simulink model "Simulink_Sfunc_Sim"  (R2022b)
settings: Solver=FixedStepAuto  StartTime=0.0  StopTime=5  FixedStep=0.01  RelTol=1e-3
values from neighbouring files (symbols this model uses):
  N = 20    [Aircraft_MPC_No_Rate_Constraints.m]    (also in Aircraft_MPC_v1.m = 100)
  nu = model.u.rows()    [Aircraft_MPC_No_Rate_Constraints.m]    (also in Aircraft_MPC_v1.m; get_aircraft_model.m = 4)
  u_max = [20000; 20000; 1700; 1700]    [Aircraft_MPC_No_Rate_Constraints.m]    (also in Aircraft_MPC_v1.m = [1000; 1000; 150; 150])
  u_min = [0; 0; 1500; 1500]    [Aircraft_MPC_No_Rate_Constraints.m]    (also in Aircraft_MPC_v1.m = [-1000; -1000; -150; -150])
  x0 = x_sim(:,i)    [Aircraft_MPC_No_Rate_Constraints.m]    (also in Aircraft_MPC_v1.m)
  x_max = [200; 200; 200; 200; 200; 200; 200; 200; 200; 200]    [Aircraft_MPC_No_Rate_Constraints.m]    (also in Aircraft_MPC_v1.m = [200; 200; 200; 200; 200; 200; 200; 200; 200; 200; 20000; 20)
  x_min = [-200; -200; -200; -200; -200; -200; -200; -200; -200; -200]    [Aircraft_MPC_No_Rate_Constraints.m]    (also in Aircraft_MPC_v1.m = [-200; -200; -200; -200; -200; -200; -200; -200; -200; -200;)
  yref = [0; 0; 0 ... (first row only)    [Aircraft_MPC_No_Rate_Constraints.m]    (also in Aircraft_MPC_v1.m = [0; 1; 1)
  yref_e = yref(1:nx)    [Aircraft_MPC_No_Rate_Constraints.m]    (also in Aircraft_MPC_v1.m)
settings Model: Creator=marcv  LastModifiedBy=marcv

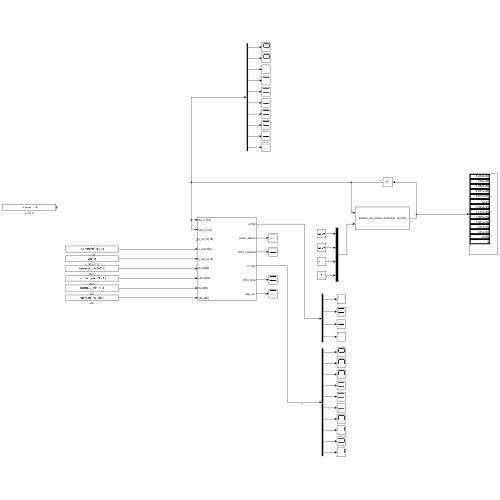
[thumbnail: Simulink's stored preview of the top-level diagram]
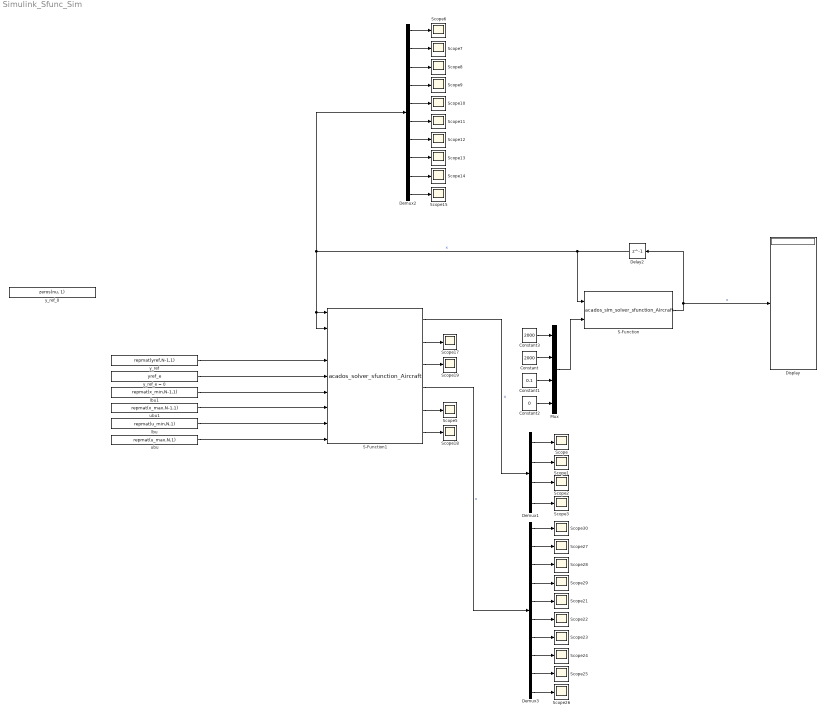
== system Simulink_Sfunc_Sim ==
  Constant : Constant  Value=2000
  Constant1 : Constant  Value=0.1
  Constant2 : Constant  Value=0
  Constant3 : Constant  Value=2000
  Delay2 : Delay  DelayLength=1  InitialCondition=x0
  Demux1 : Demux
  Demux2 : Demux  Outputs=10
  Demux3 : Demux  Outputs=10
  Display : Display
  Mux : Mux
  S-Function : S-Function  FunctionName=acados_sim_solver_sfunction_Aircraft  SFunctionDeploymentMode=off  EnableBusSupport=off
  S-Function1 : S-Function  FunctionName=acados_solver_sfunction_Aircraft  SFunctionDeploymentMode=off  EnableBusSupport=off
      mask Display:
      | % from the make_sfun file
      | global sfun_input_names sfun_output_names
      | for i = 1:length(sfun_input_names)
      | 	port_label('input', i, sfun_input_names{i})
      | end
      | for i = 1:length(sfun_output_names)
      | 	port_label('output', i, sfun_output_names{i})
      | end
  Scope{,1..3,5..15,17..19,21..30} (28 alike) : Scope
  lbu : Constant  Value=repmat(u_min,N,1)
  lbu1 : Constant  Value=repmat(x_min,N-1,1)
  ubu : Constant  Value=repmat(u_max,N,1)
  ubu1 : Constant  Value=repmat(x_max,N-1,1)
  y_ref : Constant  Value=repmat(yref,N-1,1)
  y_ref_0 : Constant  Value=zeros(nu, 1)
  y_ref_e = 0 : Constant  Value=yref_e
  wires:
  S-Function1/1 -> Demux1/1  "u"
  y_ref/1 -> S-Function1/4
  y_ref_e = 0/1 -> S-Function1/5
  lbu1/1 -> S-Function1/6
  ubu1/1 -> S-Function1/7
  Demux1/4 -> Scope3/1
  Demux1/3 -> Scope2/1
  Demux1/2 -> Scope1/1
  Demux1/1 -> Scope/1
  S-Function1/5 -> Scope5/1
  Demux2/4 -> Scope9/1
  Demux2/3 -> Scope8/1
  Demux2/1 -> Scope6/1
  Demux2/2 -> Scope7/1
  Demux2/10 -> Scope15/1
  Demux2/9 -> Scope14/1
  Demux2/8 -> Scope13/1
  Demux2/7 -> Scope12/1
  Demux2/6 -> Scope11/1
  Demux2/5 -> Scope10/1
  S-Function1/2 -> Scope17/1
  S-Function1/3 -> Scope19/1
  S-Function1/6 -> Scope18/1
  Demux3/6 -> Scope22/1
  S-Function1/4 -> Demux3/1  "x"
  Demux3/5 -> Scope21/1
  Demux3/9 -> Scope25/1
  Demux3/8 -> Scope24/1
  Demux3/3 -> Scope28/1
  Demux3/7 -> Scope23/1
  Demux3/4 -> Scope29/1
  Demux3/10 -> Scope26/1
  Demux3/1 -> Scope30/1
  Demux3/2 -> Scope27/1
  S-Function/1 -> Delay2/1, Display/1  "x"
  Delay2/1 -> Demux2/1, S-Function1/2, S-Function1/1, S-Function/1  "x"
  lbu/1 -> S-Function1/8
  ubu/1 -> S-Function1/9
  Constant3/1 -> Mux/1
  Constant/1 -> Mux/2
  Constant1/1 -> Mux/3
  Constant2/1 -> Mux/4
  Mux/1 -> S-Function/2
